simulink model "ZR_ControlsArchitecture"  (R2024b)
settings: Solver=VariableStepAuto  StartTime=0.0  StopTime=10.0  RelTol=1e-3
settings Model: Creator=ATuck  LastModifiedBy=ATuck

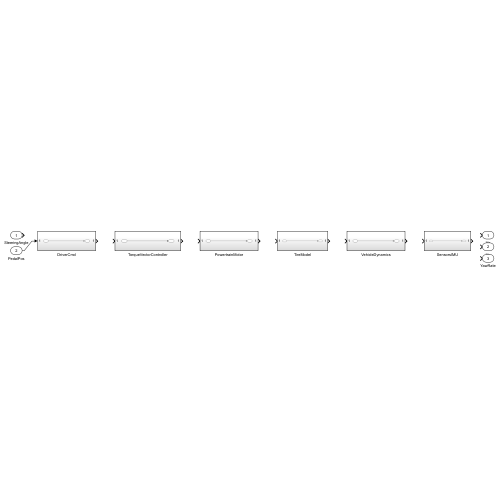
[thumbnail: Simulink's stored preview of the top-level diagram]
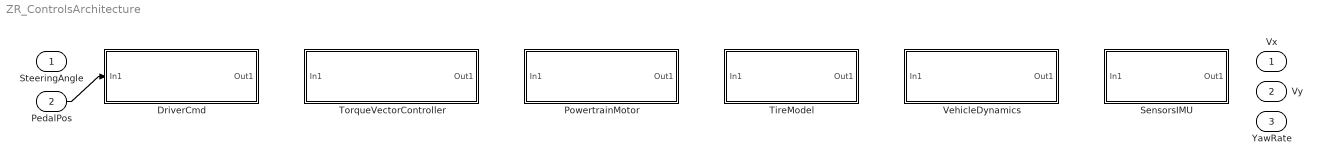
== system ZR_ControlsArchitecture ==
  SteeringAngle : Inport
  PedalPos : Inport  Port=2
  DriverCmd : Subsystem
  PowertrainMotor : Subsystem
  SensorsIMU : Subsystem
  TireModel : Subsystem
  TorqueVectorController : Subsystem
  VehicleDynamics : Subsystem
  Vx : Outport
  Vy : Outport  Port=2
  YawRate : Outport  Port=3
  wires:
  PedalPos/1 -> DriverCmd/1(In1)

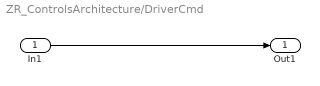
== system ZR_ControlsArchitecture/DriverCmd ==
  In1 : Inport
  Out1 : Outport
  wires:
  In1/1 -> Out1/1

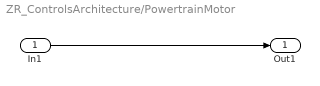
== system ZR_ControlsArchitecture/PowertrainMotor ==
  In1 : Inport
  Out1 : Outport
  wires:
  In1/1 -> Out1/1

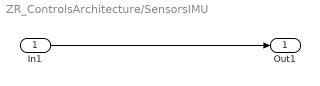
== system ZR_ControlsArchitecture/SensorsIMU ==
  In1 : Inport
  Out1 : Outport
  wires:
  In1/1 -> Out1/1

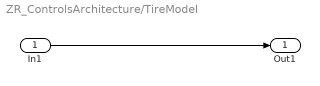
== system ZR_ControlsArchitecture/TireModel ==
  In1 : Inport
  Out1 : Outport
  wires:
  In1/1 -> Out1/1

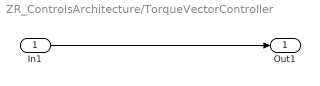
== system ZR_ControlsArchitecture/TorqueVectorController ==
  In1 : Inport
  Out1 : Outport
  wires:
  In1/1 -> Out1/1

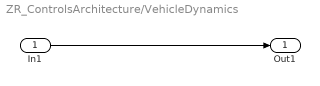
== system ZR_ControlsArchitecture/VehicleDynamics ==
  In1 : Inport
  Out1 : Outport
  wires:
  In1/1 -> Out1/1
